simulink library "INT_CoPT_TrqLeadCoord"  (R2016b)
settings: Solver=VariableStepAuto  StartTime=0.0  StopTime=10.0  RelTol=1e-3
settings Model: Creator=bianxuyin  LastModifiedBy=bianxuyin

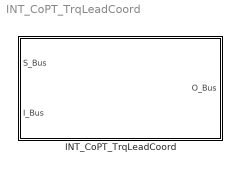
== system INT_CoPT_TrqLeadCoord ==
  INT_CoPT_TrqLeadCoord : Subsystem

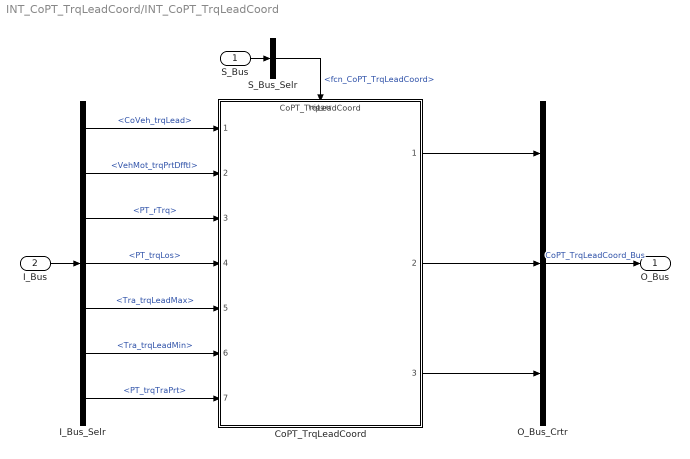
== system INT_CoPT_TrqLeadCoord/INT_CoPT_TrqLeadCoord ==
  S_Bus : Inport
  I_Bus : Inport  Port=2
  CoPT_TrqLeadCoord : ModelReference  ModelNameDialog=CoPT_TrqLeadCoord  SimulationMode=Normal  ModelReferenceVersion=1.6  TriggerPortName=function  TriggerPortTriggerType=function-call  TriggerPortStatesWhenEnabling=held
  I_Bus_Selr : BusSelector  OutputSignals=CoVeh_trqLead,VehMot_trqPrtDfftl,PT_rTrq,PT_trqLos,Tra_trqLeadMax,Tra_trqLeadMin,PT_trqTraPrt
  O_Bus_Crtr : BusCreator  Inputs=3
  S_Bus_Selr : BusSelector  OutputSignals=fcn_CoPT_TrqLeadCoord
  O_Bus : Outport
  wires:
  S_Bus_Selr/1 -> CoPT_TrqLeadCoord/Trigger  "<fcn_CoPT_TrqLeadCoord>"
  S_Bus/1 -> S_Bus_Selr/1
  I_Bus/1 -> I_Bus_Selr/1
  I_Bus_Selr/1 -> CoPT_TrqLeadCoord/1  "<CoVeh_trqLead>"
  I_Bus_Selr/2 -> CoPT_TrqLeadCoord/2  "<VehMot_trqPrtDfftl>"
  I_Bus_Selr/3 -> CoPT_TrqLeadCoord/3  "<PT_rTrq>"
  I_Bus_Selr/4 -> CoPT_TrqLeadCoord/4  "<PT_trqLos>"
  I_Bus_Selr/5 -> CoPT_TrqLeadCoord/5  "<Tra_trqLeadMax>"
  I_Bus_Selr/6 -> CoPT_TrqLeadCoord/6  "<Tra_trqLeadMin>"
  I_Bus_Selr/7 -> CoPT_TrqLeadCoord/7  "<PT_trqTraPrt>"
  O_Bus_Crtr/1 -> O_Bus/1  "CoPT_TrqLeadCoord_Bus"
  CoPT_TrqLeadCoord/1 -> O_Bus_Crtr/1
  CoPT_TrqLeadCoord/2 -> O_Bus_Crtr/2
  CoPT_TrqLeadCoord/3 -> O_Bus_Crtr/3
